simulink model "solarpanel_fixed - 복사본"  (R2024b)
settings: Solver=VariableStepAuto  StartTime=0.0  StopTime=0.1  RelTol=1e-3
libraries: spsDiodeLib x4, spsSeriesRLCBranchLib x2, spsPVArrayLib x2, spsCurrentMeasurementLib x1, spsDCVoltageSourceLib x1, spsGroundLib x1, spsMosfetLib x1, spsVoltageMeasurementLib x1, sps_lib x1
settings Model: Creator=psybe  LastModifiedBy=psybe

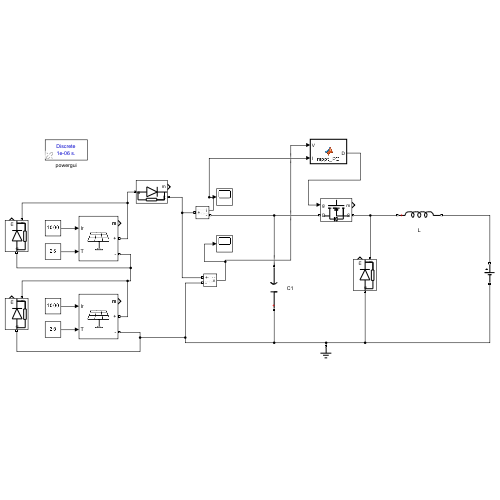
[thumbnail: Simulink's stored preview of the top-level diagram]
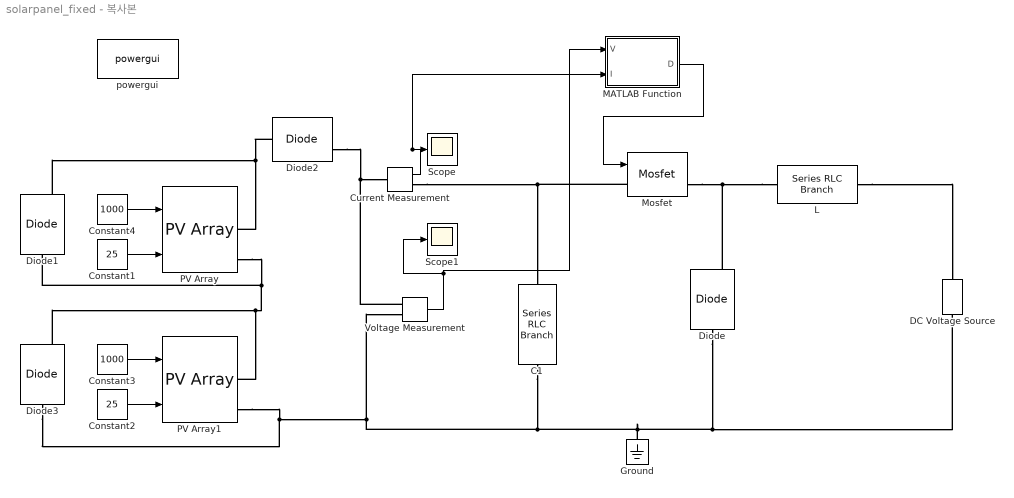
== system solarpanel_fixed - 복사본 ==
  C1 : spsSeriesRLCBranchLib/Series RLC Branch  LConnTagsString=__new0  RConnTagsString=__new0  BranchType=C  Resistance=1e-3  Inductance=1e-3  SetiL0=off  InitialCurrent=0  Capacitance=100e-6  Setx0=off  InitialVoltage=0  Measurements=None
  Constant1 : Constant  Value=25
  Constant2 : Constant  Value=25
  Constant3 : Constant  Value=1000
  Constant4 : Constant  Value=1000
  Current Measurement : spsCurrentMeasurementLib/Current Measurement  PhasorSimulation=off  OutputType=Complex  PSBequivalent=0
  DC Voltage Source : spsDCVoltageSourceLib/DC Voltage Source  Amplitude=48  Measurements=None
  Diode{,1..3} (4 alike) : spsDiodeLib/Diode  Ron=0.001  Lon=0  Vf=0.8  IC=0  UseSnubber=0  Rs=500  Cs=250e-9  Measurements=on
  Ground : spsGroundLib/Ground  LConnTagsString=a
  L : spsSeriesRLCBranchLib/Series RLC Branch  LConnTagsString=__new0  RConnTagsString=__new0  BranchType=L  Resistance=1  Inductance=150e-6  SetiL0=off  InitialCurrent=0  Capacitance=1e-6  Setx0=off  InitialVoltage=0  Measurements=None
  MATLAB Function : MATLAB Function  TreatAsAtomicUnit=on
  Mosfet : spsMosfetLib/Mosfet  Ron=0.1  Lon=0  Rd=0.01  Vfd=0  IC=0  Rs=1e5  Cs=inf  Measurements=on
  PV Array : spsPVArrayLib/PV Array  Npar=1  Nser=1  PlotType=array @ 1000 W/m2 & specified temperatures  S_vec="[ 1000  500  100 ]"  Temp_C_vec="[ 45 25  ]"  ModuleName=User-defined  PlotWhenSelected=off  Pm=213.15  Ncell=60  Voc=36.3  Isc=7.84  Vm=29  Im=7.35  beta_Voc_pc=-0.36099  alpha_Isc_pc=0.102  beta_Voc=-0.13104  alpha_Isc=0.0079968  IL=7.8654  I0=2.9273e-10  nI=0.98119  Rsh=313.0553  Rs=0.39381  RobustModel=off  RobustCellTemperature=313.3991  BAL=on  Tc=1e-6  Tfilter=5e-5
  PV Array1 : spsPVArrayLib/PV Array  Npar=1  Nser=1  PlotType=array @ 1000 W/m2 & specified temperatures  S_vec="[ 1000  500  100 ]"  Temp_C_vec="[ 45 25  ]"  ModuleName=User-defined  PlotWhenSelected=off  Pm=213.15  Ncell=60  Voc=36.3  Isc=7.84  Vm=29  Im=7.35  beta_Voc_pc=-0.36099  alpha_Isc_pc=0.102  beta_Voc=-0.13104  alpha_Isc=0.0079968  IL=7.8654  I0=2.9273e-10  nI=0.98119  Rsh=313.0553  Rs=0.39381  RobustModel=off  RobustCellTemperature=313.3991  BAL=on  Tc=1e-6  Tfilter=5e-5
  Scope : Scope
  Scope1 : Scope
  Voltage Measurement : spsVoltageMeasurementLib/Voltage Measurement  PhasorSimulation=off  OutputType=Complex  PSBequivalent=0
  powergui : sps_lib/powergui  Priority=1  SimulationMode=Discrete  SampleTime=1e-6  frequency=60  Iterations=50  frequencyindice=0  Pbase=100e6  ErrMax=1e-4  UnitsV=kV  UnitsW=MW  buscounter=0  FunctionMessages=off  echomessages=off  EnableUseOfTLC=off  CurrentSourceSwitches=off  DisableSnubberDevices=off  DisableRonSwitches=off  DisableVfSwitches=off  DisplayEquations=off  AutomaticDiscreteSolvers=off  SolverType=Tustin/Backward Euler (TBE)  Interpol=off  ExternalGateDelay=off  methode=off  Ts=100  x0status=blocks  SPID=on  SwTol=0  HookPort=off  NonlinearTolerance=1e-4  nMaxIteration=100  ContinueOnMaxIteration=off  RestoreLinks=warning  ResistiveCurrentMeasurement=off  Frange=[0:2:500]  Ylog=off  Xlog=on  ShowGrid=off  save=off  variable=ZData  structure=0  ZoomFFT=off  StartTime=0.0  cycles=1  DisplayStyle=1  fundamental=60  FreqAxis=off  MaxFrequency=1000  frequencyindicesteady=1  RmsSteady=1  display=off
  wires:
  MATLAB Function/1(D) -> Mosfet/1
  Constant1/1 -> PV Array/2
  Constant4/1 -> PV Array/1
  Current Measurement/1 -> MATLAB Function/2(I), Scope/1
  Voltage Measurement/1 -> MATLAB Function/1(V), Scope1/1
  Constant3/1 -> PV Array1/1
  Constant2/1 -> PV Array1/2
  connections:
  C1/LConn1 -- Diode3/LConn1 -- PV Array1/RConn2 -- Voltage Measurement/LConn2 -- Ground/LConn1 -- Diode/LConn1 -- DC Voltage Source/LConn1
  Mosfet/LConn1 -- Current Measurement/RConn1 -- C1/RConn1
  Voltage Measurement/LConn1 -- Diode2/RConn1 -- Current Measurement/LConn1
  L/LConn1 -- Mosfet/RConn1 -- Diode/RConn1
  L/RConn1 -- DC Voltage Source/RConn1
  Diode2/LConn1 -- Diode1/RConn1 -- PV Array/RConn1
  PV Array1/RConn1 -- PV Array/RConn2 -- Diode1/LConn1 -- Diode3/RConn1

== matlab function solarpanel_fixed - 복사본/MATLAB Function ==
  data: V input; D output; I input
function D = mppt_PO(V, I)
% P&O MPPT Algorithm for Buck Converter

% 과거의 전압, 전력, 듀티비를 기억하기 위한 변수 선언
persistent V_old P_old D_old;

% 맨 처음 0초일 때 초기값 세팅
if isempty(V_old)
    V_old = 0; 
    P_old = 0; 
    D_old = 0.5; % 듀티비 50%에서 시작
end

delta_D = 0.005; % 발걸음 크기 (한 번에 듀티비를 얼마나 바꿀지)
P = V * I;       % 현재 전력 계산 ($P = V \times I$)

% 산 정상 찾아가기 로직 (전력이 올랐는가?)
if (P - P_old) > 0
    if (V - V_old) > 0
        D = D_old - delta_D; % 벅 컨버터는 V를 높이려면 D를 줄여야 함
    else
        D = D_old + delta_D;
    end
else % 전력이 떨어졌는가? (방향 반대로!)
    if (V - V_old) > 0
        D = D_old + delta_D; 
    else
        D = D_old - delta_D;
    end
end

% 듀티비가 미쳐 날뛰지 않게 한계선 설정 (10% ~ 90%)
if D > 0.9
    D = 0.9; 
end
if D < 0.1
    D = 0.1; 
end

% 다음 계산을 위해 현재 값을 기억에 저장
V_old = V;
P_old = P;
D_old = D;

end
